simulink model "NULMPC_RAS"  (R2024a)
settings: Solver=FixedStepAuto  StartTime=0.0  StopTime=10  FixedStep=Ts  RelTol=1e-3
values from neighbouring files (symbols this model uses):
  alpha_o = 1/(ms) + 1/(mu)    [nulmpc.m]
  bs = 7.5    [initparams.m]
  bus = 5    [initparams.m]
  delta_Fc_max = 1000*Ts    (= 10)    [initparams.m]
  delta_Fc_min = -1000*Ts    (= -10)    [initparams.m]
  E = 1    [nmpc.m]    (also in nulmpc.m = 5)
  Fc_max = 15    [initparams.m]
  Fc_min = -15    [initparams.m]
  Hc = 1    [initparams.m]
  ks = 900    [initparams.m]
  kus = kt    (= 2500)    [initparams.m]
  ms = 2.45    [initparams.m]
  mus = mu    (= 1)    [initparams.m]
  n_max = 0.05    [initparams.m]
  n_min = -0.05    [initparams.m]
  Q_n = 10000    [nmpc.m]    (also in nulmpc.m = 1000)
  Q_ndot = 100    [nmpc.m]    (also in nulmpc.m = 5)
  R = 10    [nmpc.m]    (also in nulmpc.m)
  Ts = 0.01    [initparams.m]
  z1_dot_init = 0    [initparams.m]
  z1_init = 0.005    [initparams.m]
  z2_dot_init = 0    [initparams.m]
  z2_init = 0    [initparams.m]
libraries: simulink x1, mpclib x1
settings Model: Creator=aidan  LastModifiedBy=aidan
settings DebuggingCC: UnderSpecifiedDimensionMsg=warning
settings HardwareCC: ProdHWDeviceType=AMD->x86-64 (Windows64)

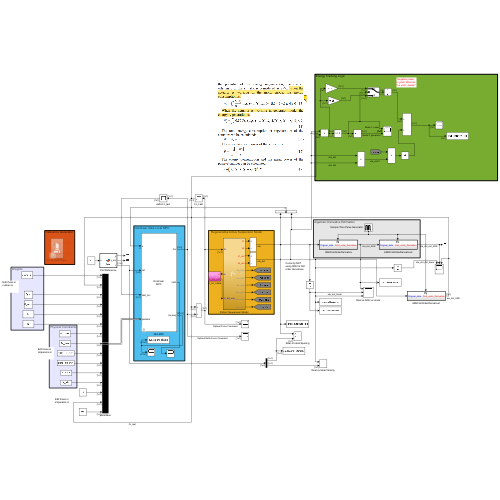
[thumbnail: Simulink's stored preview of the top-level diagram]
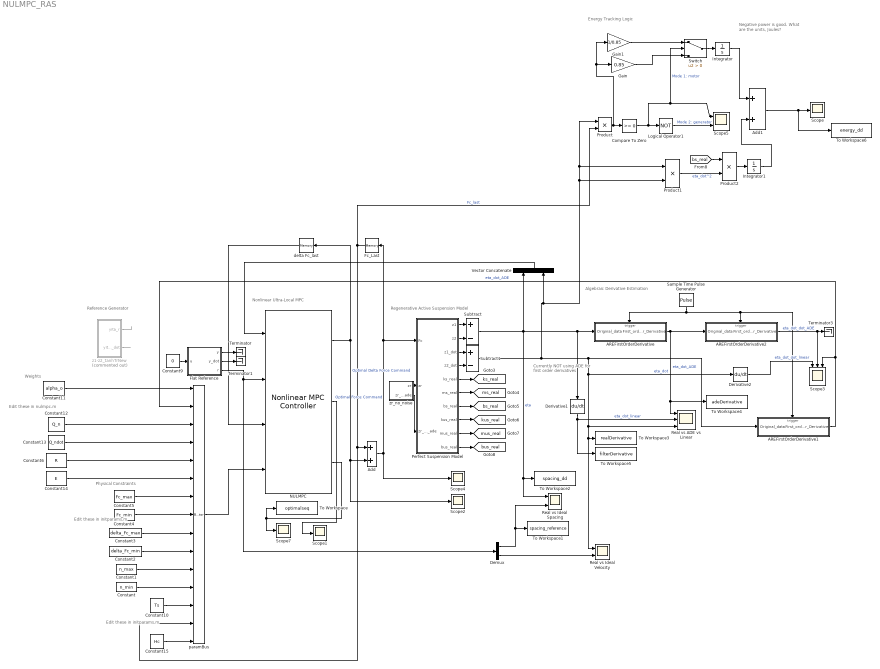
== system NULMPC_RAS ==
  note: Edit these in nulmpc.m
  note: Currently NOT using ADE for first order derivatives
  note: Nonlinear Ultra-Local MPC
  note: Energy Tracking Logic
  note: Regenerative Active Suspension Model
  note: Reference Generator
  note: Algebraic Derivative Estimation
  note: Weights
  note: Physical Constraints
  note: Negative power is good. What are the units, Joules?
  note: Edit these in initparams.m
  note: Edit these in initparams.m
  AREFirstOrderDerivative : Subsystem  TreatAsAtomicUnit=on
  AREFirstOrderDerivative1 : Subsystem  TreatAsAtomicUnit=on
  AREFirstOrderDerivative2 : Subsystem  TreatAsAtomicUnit=on
  Add : Sum
  Add1 : Sum
  Compare To Zero : simulink/Logic and Bit Operations/Compare To Zero  relop=>=  OutDataTypeStr=boolean
  Constant : Constant  Value=n_min
  Constant1 : Constant  Value=n_max
  Constant10 : Constant  Value=Ts
  Constant11 : Constant  Value=alpha_o
  Constant12 : Constant  Value=Q_n
  Constant13 : Constant  Value=Q_ndot
  Constant14 : Constant  Value=E
  Constant15 : Constant  Value=Hc
  Constant2 : Constant  Value=delta_Fc_min
  Constant3 : Constant  Value=delta_Fc_max
  Constant4 : Constant  Value=Fc_min
  Constant5 : Constant  Value=Fc_max
  Constant6 : Constant  Value=R
  Constant9 : Constant  Value=0
  Demux : Demux  Outputs=2
  Derivative1 : Derivative
  Derivative2 : Derivative
  Fc_Last : Memory  InheritSampleTime=on
  Flat Reference : MATLAB Function  TreatAsAtomicUnit=on
  Gain : Gain  Gain=0.85
  Gain1 : Gain  Gain=1/0.85
  Integrator : Integrator
  Integrator1 : Integrator
  Logical Operator1 : Logic  Operator=NOT  AllPortsSameDT=off  OutDataTypeStr=boolean
  NULMPC : mpclib/Nonlinear MPC Controller  nlmpcobj=nulmpcobj  UseObjectTs=on  UseMEX=off  md_enabled=off  mvtarget_enabled=off  param_enabled=on  cost_enabled=on  mvseq_enabled=on  stateseq_enabled=off  ovseq_enabled=off  slack_enabled=off  status_enabled=off  ov_min=off  ov_max=off  mv_min=off  mv_max=off  mvrate_min=off  mvrate_max=off  state_min=off  state_max=off  ov_weight=off  mv_weight=off  mvrate_weight=off  ecr_weight=off  nlp_initialize=off
  Perfect Suspension Model : Subsystem
  Product : Product
  Product1 : Product
  Product2 : Product
  Real vs ADE vs Linear : Scope  NumInputPorts=3
  Real vs Ideal Spacing : Scope  NumInputPorts=2
  Real vs Ideal Velocity : Scope  NumInputPorts=2
  Sample Time Pulse Generator : DiscretePulseGenerator  PulseType=Time based  Period=Ts*2  PulseWidth=50
  Scope{,1..2,4,7} (5 alike) : Scope
  Scope3 : Scope  NumInputPorts=3
  Scope5 : Scope  NumInputPorts=2
  Subtract : Sum  Inputs=+-
  Subtract1 : Sum  Inputs=+-
  Switch : Switch  Criteria=u2 > Threshold  SaturateOnIntegerOverflow=off  InputSameDT=off
  Terminator : Terminator
  Terminator1 : Terminator
  Terminator3 : Terminator
  To Workspace : ToWorkspace  VariableName=optimalseq  SaveFormat=Timeseries  SampleTime=-1
  To Workspace1 : ToWorkspace  VariableName=spacing_reference  SaveFormat=Timeseries  SampleTime=-1
  To Workspace2 : ToWorkspace  VariableName=spacing_dd  SaveFormat=Timeseries  SampleTime=-1
  To Workspace3 : ToWorkspace  VariableName=realDerivative  SaveFormat=Timeseries  SampleTime=-1
  To Workspace4 : ToWorkspace  VariableName=adeDerivative  SaveFormat=Timeseries  SampleTime=-1
  To Workspace5 : ToWorkspace  VariableName=filterDerivative  SaveFormat=Timeseries  SampleTime=-1
  To Workspace6 : ToWorkspace  VariableName=energy_dd  SaveFormat=Timeseries  SampleTime=-1
  Vector Concatenate : Concatenate
  delta Fc_last : Memory  InheritSampleTime=on
  paramBus : BusCreator  Inputs=15  OutDataTypeStr=Bus: paramBus  NonVirtualBus=on
      settings: InheritFromInputs=off
  "z1-z2_tanhTrNew " : Subsystem  Commented=on
  zr_no_noise : Subsystem
  tag scope: bs_real=global, bus_real=global, ks_real=global, kus_real=global, ms_real=global, mus_real=global
  wires:
  Constant5/1 -> paramBus/7
  Constant4/1 -> paramBus/8
  Constant3/1 -> paramBus/9
  Constant2/1 -> paramBus/10
  Constant1/1 -> paramBus/11
  Constant/1 -> paramBus/12
  Constant6/1 -> paramBus/5
  NULMPC/1 -> delta Fc_last/1, Scope2/1, Add/2  "Optimal Delta Force Command"
  Perfect Suspension Model/5(ks_real) -> [ks_real]
  Perfect Suspension Model/6(ms_real) -> [ms_real]
  Perfect Suspension Model/7(bs_real) -> [bs_real]
  Perfect Suspension Model/8(kus_real) -> [kus_real]
  Perfect Suspension Model/9(mus_real) -> [mus_real]
  Perfect Suspension Model/10(bus_real) -> [bus_real]
  Perfect Suspension Model/3(z1_dot) -> Subtract1/1
  Perfect Suspension Model/4(z2_dot) -> Subtract1/2
  Perfect Suspension Model/2(z2) -> Subtract/2
  Perfect Suspension Model/1(z1) -> Subtract/1
  Sample Time Pulse Generator/1 -> AREFirstOrderDerivative1/Trigger, AREFirstOrderDerivative2/Trigger, AREFirstOrderDerivative/Trigger
  Fc_Last/1 -> paramBus/14, Add/1, Product/2  "Fc_last"
  AREFirstOrderDerivative/1(First_order_Derivative) -> AREFirstOrderDerivative2/1(Original_data), To Workspace4/1, Real vs ADE vs Linear/1  "eta_dot_ADE"
  AREFirstOrderDerivative2/1(First_order_Derivative) -> Scope3/2, Terminator3/1  "eta_dot_dot_ADE"
  Vector Concatenate/1 -> NULMPC/1
  Constant13/1 -> paramBus/4
  Constant12/1 -> paramBus/3
  Add/1 -> Scope4/1, Perfect Suspension Model/1(Fc), Fc_Last/1  "Optimal Force Command"
  Derivative1/1 -> To Workspace5/1, Real vs ADE vs Linear/2  "eta_dot_linear"
  Derivative2/1 -> Scope3/1  "eta_dot_dot_linear"
  Subtract/1 -> Real vs Ideal Spacing/1, To Workspace2/1, Vector Concatenate/1, AREFirstOrderDerivative/1(Original_data), Derivative1/1  "eta"
  zr_no_noise/1(zr) -> Perfect Suspension Model/2(zr)
  Constant9/1 -> Flat Reference/1(u)
  "z1-z2_tanhTrNew "/2(yitar_dot) -> ?
  "z1-z2_tanhTrNew "/1(yita_r) -> ?
  Flat Reference/2(y_dot) -> Terminator1/1
  Flat Reference/1(y) -> Terminator/1
  paramBus/1 -> NULMPC/4
  Constant11/1 -> paramBus/1
  Constant14/1 -> paramBus/6
  delta Fc_last/1 -> NULMPC/3
  Constant10/1 -> paramBus/13
  Flat Reference/3(r) -> Demux/1, NULMPC/2
  Constant15/1 -> paramBus/15
  Demux/1 -> Real vs Ideal Spacing/2, To Workspace1/1
  Demux/2 -> Real vs Ideal Velocity/2
  Logical Operator1/1 -> Scope5/2  "Mode 2: generator"
  Compare To Zero/1 -> Switch/2, Scope5/1, Logical Operator1/1  "Mode 1: motor"
  NULMPC/2 -> Scope1/1
  NULMPC/3 -> Scope7/1, To Workspace/1
  Product/1 -> Gain/1, Gain1/1, Compare To Zero/1
  Switch/1 -> Integrator/1
  Gain/1 -> Switch/3
  Gain1/1 -> Switch/1
  AREFirstOrderDerivative1/1(First_order_Derivative) -> paramBus/2, Scope3/3  "eta_dot_ADE"
  zr_no_noise/2(zr_dot_ade) -> Perfect Suspension Model/3(zr_dot_ade)
  Subtract1/1 -> Vector Concatenate/2, Product/1, Product1/1, Product1/2, AREFirstOrderDerivative1/1(Original_data), Real vs Ideal Velocity/1, To Workspace3/1, Real vs ADE vs Linear/3, Derivative2/1  "eta_dot"
  Integrator1/1 -> Add1/2
  Product2/1 -> Integrator1/1
  Product1/1 -> Product2/2  "eta_dot^2"
  [bs_real] -> Product2/1
  Integrator/1 -> Add1/1
  Add1/1 -> Scope/1, To Workspace6/1

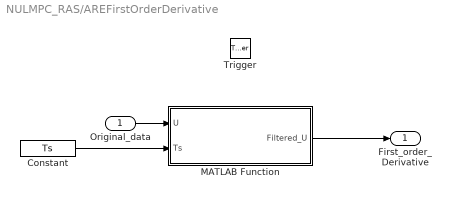
== system NULMPC_RAS/AREFirstOrderDerivative ==
  Original_data : Inport
  Trigger : TriggerPort  TriggerType=either  VariantControl=Variant  ZeroCross=off  PortDimensions=1
  Constant : Constant  Value=Ts
  MATLAB Function : MATLAB Function  TreatAsAtomicUnit=on
  First_order_Derivative : Outport  VectorParamsAs1DForOutWhenUnconnected=off
  wires:
  Constant/1 -> MATLAB Function/2(Ts)
  MATLAB Function/1(Filtered_U) -> First_order_Derivative/1
  Original_data/1 -> MATLAB Function/1(U)

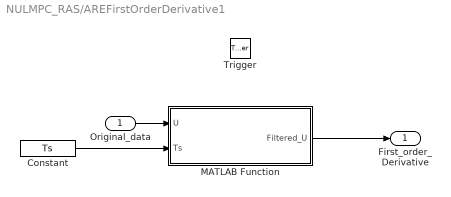
== system NULMPC_RAS/AREFirstOrderDerivative1 ==
  Original_data : Inport
  Trigger : TriggerPort  TriggerType=either  VariantControl=Variant  ZeroCross=off  PortDimensions=1
  Constant : Constant  Value=Ts
  MATLAB Function : MATLAB Function  TreatAsAtomicUnit=on
  First_order_Derivative : Outport  VectorParamsAs1DForOutWhenUnconnected=off
  wires:
  Constant/1 -> MATLAB Function/2(Ts)
  MATLAB Function/1(Filtered_U) -> First_order_Derivative/1
  Original_data/1 -> MATLAB Function/1(U)

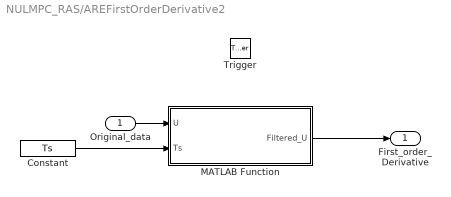
== system NULMPC_RAS/AREFirstOrderDerivative2 ==
  Original_data : Inport
  Trigger : TriggerPort  TriggerType=either  VariantControl=Variant  ZeroCross=off  PortDimensions=1
  Constant : Constant  Value=Ts
  MATLAB Function : MATLAB Function  TreatAsAtomicUnit=on
  First_order_Derivative : Outport  VectorParamsAs1DForOutWhenUnconnected=off
  wires:
  Constant/1 -> MATLAB Function/2(Ts)
  MATLAB Function/1(Filtered_U) -> First_order_Derivative/1
  Original_data/1 -> MATLAB Function/1(U)

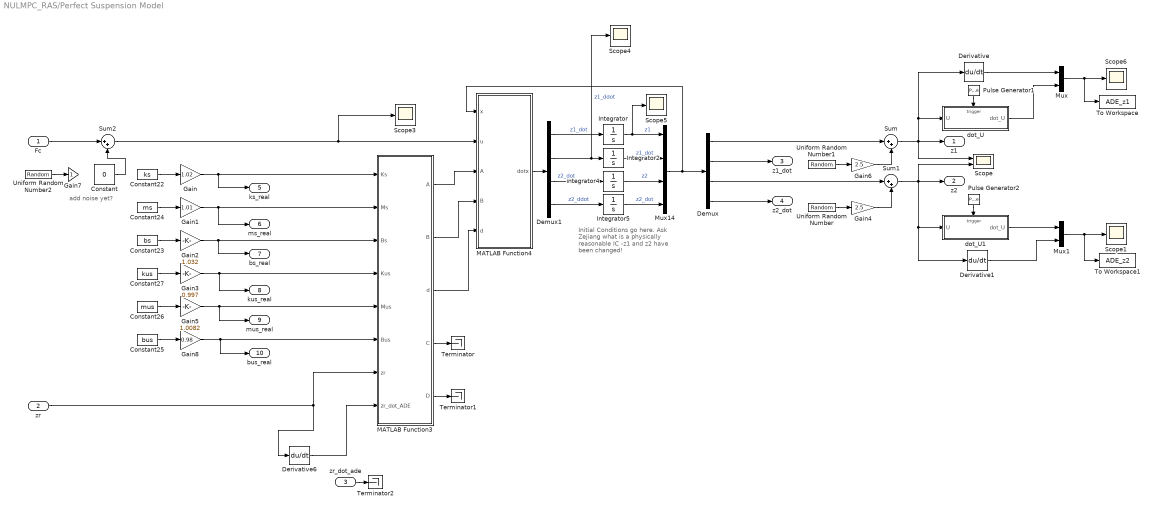
== system NULMPC_RAS/Perfect Suspension Model ==
  note: Initial Conditions go here. Ask Zejiang what is a physically reasonable IC
      |
      | -z1 and z2 have been changed!
  note: add noise yet?
  Fc : Inport
  zr : Inport  Port=2
  zr_dot_ade : Inport  Port=3
  Constant : Constant  Value=0
  Constant22 : Constant  Value=ks
  Constant23 : Constant  Value=bs
  Constant24 : Constant  Value=ms
  Constant25 : Constant  Value=bus
  Constant26 : Constant  Value=mus
  Constant27 : Constant  Value=kus
  Demux : Demux
  Demux1 : Demux
  Derivative : Derivative
  Derivative1 : Derivative
  Derivative6 : Derivative
  Gain : Gain  Gain=1.02
  Gain1 : Gain  Gain=1.01
  Gain2 : Gain  Gain=1.032
  Gain3 : Gain  Gain=0.997
  Gain4 : Gain  Gain=2.5
  Gain5 : Gain  Gain=1.0082
  Gain6 : Gain  Gain=2.5
  Gain7 : Gain
  Gain8 : Gain  Gain=0.98
  Integrator : Integrator  InitialCondition=z1_init
  Integrator2 : Integrator  InitialCondition=z1_dot_init
  Integrator4 : Integrator  InitialCondition=z2_init
  Integrator5 : Integrator  InitialCondition=z2_dot_init
  MATLAB Function3 : MATLAB Function  TreatAsAtomicUnit=on
  MATLAB Function4 : MATLAB Function  TreatAsAtomicUnit=on
  Mux : Mux  Inputs=2
  Mux1 : Mux  Inputs=2
  Mux14 : Mux
  Pulse Generator1 : DiscretePulseGenerator  PulseType=Time based  Period=Ts*2  PulseWidth=50
  Pulse Generator2 : DiscretePulseGenerator  PulseType=Time based  Period=Ts*2  PulseWidth=50
  Scope : Scope  NumInputPorts=2
  Scope{1,3..6} (5 alike) : Scope
  Sum : Sum  Inputs=|++
  Sum1 : Sum  Inputs=|++
  Sum2 : Sum  Inputs=|++
  Terminator : Terminator
  Terminator1 : Terminator
  Terminator2 : Terminator
  To Workspace : ToWorkspace  VariableName=ADE_z1  SampleTime=-1
  To Workspace1 : ToWorkspace  VariableName=ADE_z2  SampleTime=-1
  Uniform Random Number : UniformRandomNumber  Minimum=-1e-6  Maximum=1e-6  Seed=244334  SampleTime=Ts
  Uniform Random Number1 : UniformRandomNumber  Minimum=-1e-6  Maximum=1e-6  Seed=7  SampleTime=Ts
  Uniform Random Number2 : UniformRandomNumber  Minimum=-5e-3  Maximum=5e-3  Seed=89757  SampleTime=Ts
  dot_U : Subsystem  TreatAsAtomicUnit=on
  dot_U1 : Subsystem  TreatAsAtomicUnit=on
  z1 : Outport
  z2 : Outport  Port=2
  z1_dot : Outport  Port=3
  z2_dot : Outport  Port=4
  ks_real : Outport  Port=5
  ms_real : Outport  Port=6
  bs_real : Outport  Port=7
  kus_real : Outport  Port=8
  mus_real : Outport  Port=9
  bus_real : Outport  Port=10
  wires:
  Constant23/1 -> Gain2/1
  MATLAB Function3/4(C) -> Terminator/1
  Demux1/1 -> Integrator/1  "z1_dot"
  zr/1 -> MATLAB Function3/7(zr), Derivative6/1
  Integrator5/1 -> Mux14/4  "z2_dot"
  Demux1/2 -> Scope4/1, Integrator2/1  "z1_ddot"
  Gain2/1 -> bs_real/1, MATLAB Function3/3(Bs)
  Constant27/1 -> Gain3/1
  Gain3/1 -> kus_real/1, MATLAB Function3/4(Kus)
  Constant24/1 -> Gain1/1
  Constant25/1 -> Gain8/1
  Demux1/4 -> Integrator5/1  "z2_ddot"
  MATLAB Function4/1(dotx) -> Demux1/1
  Integrator4/1 -> Mux14/3  "z2"
  Integrator/1 -> Scope5/1, Mux14/1  "z1"
  Constant26/1 -> Gain5/1
  Gain8/1 -> bus_real/1, MATLAB Function3/6(Bus)
  MATLAB Function3/2(B) -> MATLAB Function4/4(B)
  Constant22/1 -> Gain/1
  Demux1/3 -> Integrator4/1  "z2_dot"
  Gain5/1 -> mus_real/1, MATLAB Function3/5(Mus)
  MATLAB Function3/5(D) -> Terminator1/1
  Integrator2/1 -> Mux14/2  "z1_dot"
  Gain1/1 -> ms_real/1, MATLAB Function3/2(Ms)
  Gain/1 -> ks_real/1, MATLAB Function3/1(Ks)
  MATLAB Function3/1(A) -> MATLAB Function4/3(A)
  Mux14/1 -> Demux/1, MATLAB Function4/1(x)
  MATLAB Function3/3(d) -> MATLAB Function4/5(d)
  Demux/2 -> z1_dot/1
  Demux/4 -> z2_dot/1
  Gain4/1 -> Sum1/2
  Uniform Random Number/1 -> Gain4/1
  Sum/1 -> Scope/1, Derivative/1, dot_U/1(U), z1/1
  Demux/1 -> Sum/1
  Demux/3 -> Sum1/1
  Uniform Random Number1/1 -> Gain6/1
  Gain6/1 -> Sum/2
  dot_U/1(dot_U) -> Mux/2
  Pulse Generator1/1 -> dot_U/Trigger
  Derivative/1 -> Mux/1
  Pulse Generator2/1 -> dot_U1/Trigger
  Sum1/1 -> Scope/2, Derivative1/1, dot_U1/1(U), z2/1
  dot_U1/1(dot_U) -> Mux1/1
  Derivative1/1 -> Mux1/2
  Sum2/1 -> Scope3/1, MATLAB Function4/2(u)
  Fc/1 -> Sum2/1
  Uniform Random Number2/1 -> Gain7/1
  Mux/1 -> To Workspace/1, Scope6/1
  Mux1/1 -> Scope1/1, To Workspace1/1
  Constant/1 -> Sum2/2
  zr_dot_ade/1 -> Terminator2/1
  Derivative6/1 -> MATLAB Function3/8(zr_dot_ADE)

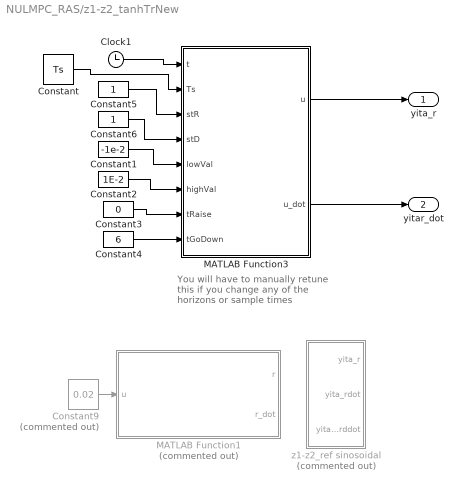
== system NULMPC_RAS/z1-z2_tanhTrNew  ==
  note: You will have to manually retune this if you change any of the horizons or sample times
  Clock1 : Clock
  Constant : Constant  Value=Ts
  Constant1 : Constant  Value=-1e-2
  Constant2 : Constant  Value=1E-2
  Constant3 : Constant  Value=0
  Constant4 : Constant  Value=6
  Constant5 : Constant
  Constant6 : Constant
  Constant9 : Constant  Commented=on  Value=0.02
  MATLAB Function1 : MATLAB Function  Commented=on  TreatAsAtomicUnit=on
  MATLAB Function3 : MATLAB Function  TreatAsAtomicUnit=on
  z1-z2_ref sinosoidal : Subsystem  Commented=on
  yita_r : Outport
  yitar_dot : Outport  Port=2
  wires:
  Constant5/1 -> MATLAB Function3/3(stR)
  Constant4/1 -> MATLAB Function3/8(tGoDown)
  Constant3/1 -> MATLAB Function3/7(tRaise)
  Clock1/1 -> MATLAB Function3/1(t)
  Constant6/1 -> MATLAB Function3/4(stD)
  MATLAB Function3/1(u) -> yita_r/1
  Constant1/1 -> MATLAB Function3/5(lowVal)
  Constant2/1 -> MATLAB Function3/6(highVal)
  MATLAB Function3/2(u_dot) -> yitar_dot/1
  Constant/1 -> MATLAB Function3/2(Ts)
  Constant9/1 -> MATLAB Function1/1(u)

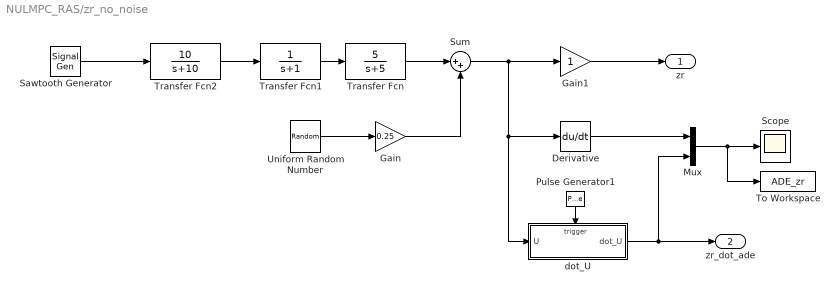
== system NULMPC_RAS/zr_no_noise ==
  Derivative : Derivative
  Gain : Gain  Gain=0.25
  Gain1 : Gain
  Mux : Mux  Inputs=2
  Pulse Generator1 : DiscretePulseGenerator  PulseType=Time based  Period=Ts*2  PulseWidth=50
  Sawtooth Generator : SignalGenerator  WaveForm=sawtooth  Amplitude=3.5e-2
  Scope : Scope
  Sum : Sum  Inputs=|++
  To Workspace : ToWorkspace  VariableName=ADE_zr  SampleTime=-1
  Transfer Fcn : TransferFcn  Numerator=[5]  Denominator=[1 5]
  Transfer Fcn1 : TransferFcn  Denominator=[1 1]
  Transfer Fcn2 : TransferFcn  Numerator=[10]  Denominator=[1 10]
  Uniform Random Number : UniformRandomNumber  Minimum=-1e-6  Maximum=1e-6  Seed=122334  SampleTime=Ts
  dot_U : Subsystem  TreatAsAtomicUnit=on
  zr : Outport
  zr_dot_ade : Outport  Port=2
  wires:
  Transfer Fcn2/1 -> Transfer Fcn1/1
  Transfer Fcn/1 -> Sum/1
  Sawtooth Generator/1 -> Transfer Fcn2/1
  Transfer Fcn1/1 -> Transfer Fcn/1
  Uniform Random Number/1 -> Gain/1
  Gain/1 -> Sum/2
  Pulse Generator1/1 -> dot_U/Trigger
  Derivative/1 -> Mux/1
  dot_U/1(dot_U) -> zr_dot_ade/1, Mux/2
  Mux/1 -> To Workspace/1, Scope/1
  Sum/1 -> dot_U/1(U), Derivative/1, Gain1/1
  Gain1/1 -> zr/1

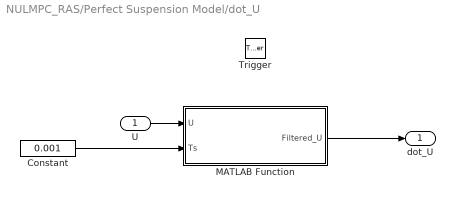
== system NULMPC_RAS/Perfect Suspension Model/dot_U ==
  U : Inport
  Trigger : TriggerPort  TriggerType=either  VariantControl=Variant  ZeroCross=off  PortDimensions=1
  Constant : Constant  Value=0.001
  MATLAB Function : MATLAB Function  TreatAsAtomicUnit=on
  dot_U : Outport  VectorParamsAs1DForOutWhenUnconnected=off
  wires:
  Constant/1 -> MATLAB Function/2(Ts)
  MATLAB Function/1(Filtered_U) -> dot_U/1
  U/1 -> MATLAB Function/1(U)

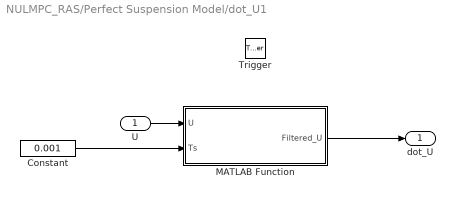
== system NULMPC_RAS/Perfect Suspension Model/dot_U1 ==
  U : Inport
  Trigger : TriggerPort  TriggerType=either  VariantControl=Variant  ZeroCross=off  PortDimensions=1
  Constant : Constant  Value=0.001
  MATLAB Function : MATLAB Function  TreatAsAtomicUnit=on
  dot_U : Outport  VectorParamsAs1DForOutWhenUnconnected=off
  wires:
  U/1 -> MATLAB Function/1(U)
  MATLAB Function/1(Filtered_U) -> dot_U/1
  Constant/1 -> MATLAB Function/2(Ts)

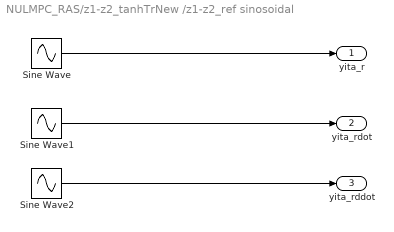
== system NULMPC_RAS/z1-z2_tanhTrNew /z1-z2_ref sinosoidal ==
  Sine Wave : Sin  Amplitude=1e-2  Frequency=2*pi/5  SampleTime=0
  Sine Wave1 : Sin  Amplitude=1e-2*2*pi/5  Frequency=2*pi/5  Phase=pi/2  SampleTime=0
  Sine Wave2 : Sin  Amplitude=-1e-2*(2*pi/5)^2  Frequency=2*pi/5  SampleTime=0
  yita_r : Outport
  yita_rdot : Outport  Port=2
  yita_rddot : Outport  Port=3
  wires:
  Sine Wave/1 -> yita_r/1
  Sine Wave1/1 -> yita_rdot/1
  Sine Wave2/1 -> yita_rddot/1

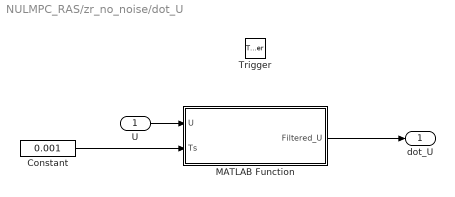
== system NULMPC_RAS/zr_no_noise/dot_U ==
  U : Inport
  Trigger : TriggerPort  TriggerType=either  VariantControl=Variant  ZeroCross=off  PortDimensions=1
  Constant : Constant  Value=0.001
  MATLAB Function : MATLAB Function  TreatAsAtomicUnit=on
  dot_U : Outport  VectorParamsAs1DForOutWhenUnconnected=off
  wires:
  Constant/1 -> MATLAB Function/2(Ts)
  MATLAB Function/1(Filtered_U) -> dot_U/1
  U/1 -> MATLAB Function/1(U)

== matlab function NULMPC_RAS/AREFirstOrderDerivative2/MATLAB Function ==
  data: U input; Filtered_U output; Ts input
function Filtered_U = buffer(U,Ts)
    N = 8; %6
    %Ts = 0.01;
    persistent y;
    if isempty(y)
        y=zeros(N+1,1);
    end

    y = [U;y(1:end-1)];
    T = Ts*N;
    P = zeros(1,N+1);
    P_alpha = P;
    for k = 1:N+1
        tao_k = (k-1)*Ts;
        P(k) = T-2*tao_k;
        if((k==1)||(k==N+1))
            P_alpha(k) = P(k)*Ts/2;
        else
            P_alpha(k) = P(k)*Ts;
        end
    end
    
    Filtered_U = P_alpha*y*6/(T^3);

end

== matlab function NULMPC_RAS/Perfect Suspension Model/MATLAB Function4 ==
  data: x input; dotx output; u input; A input; B input; d input
function dotx  = Susp_System(x, u, A, B, d)
    
    dotx = A*x + B*u + d;
    %y = C*x + D*u;
end

== matlab function NULMPC_RAS/AREFirstOrderDerivative/MATLAB Function ==
  data: U input; Filtered_U output; Ts input
function Filtered_U = buffer(U,Ts)
    % was 12
    N = 8;
    persistent y;
    if isempty(y)
        y=zeros(N+1,1);
    end

    y = [U;y(1:end-1)];
    T = Ts*N;
    P = zeros(1,N+1);
    P_alpha = P;
    for k = 1:N+1
        tao_k = (k-1)*Ts;
        P(k) = T-2*tao_k;
        if((k==1)||(k==N+1))
            P_alpha(k) = P(k)*Ts/2;
        else
            P_alpha(k) = P(k)*Ts;
        end
    end
    
    Filtered_U = P_alpha*y*6/(T^3);

end

== matlab function NULMPC_RAS/Perfect Suspension Model/MATLAB Function3 ==
  data: Ks input; A output; Ms input; Bs input; Kus input; Mus input; Bus input; zr input; zr_dot_ADE input; B output; d output; C output; D output
function [A, B, d, C, D] = Syst(Ks, Ms, Bs, Kus, Mus, Bus, zr, zr_dot_ADE)
    A = [    0,      1,             0,              0; 
        -Ks/Ms, -Bs/Ms,         Ks/Ms,          Bs/Ms; 
             0,      0,             0,              1; 
        Ks/Mus, Bs/Mus, -(Kus+Ks)/Mus, -(Bus+Bs)/Mus];
 
    
    B = [0; 1/Ms; 0; -1/Mus];
    
    
    d = [0;    0; 0;  Kus/Mus*zr + Bus/Mus*zr_dot_ADE];
   
    
    C = [    1,      0,    -1,     0;
        -Ks/Ms, -Bs/Ms, Ks/Ms, Bs/Ms];
    
    D = [0; 1/Ms];
    
    
end

== matlab function NULMPC_RAS/zr_no_noise/dot_U/MATLAB Function ==
  data: U input; Filtered_U output; Ts input
function Filtered_U = buffer(U,Ts)
    N = 10;
    %Ts = 0.001;
    persistent y;
    if isempty(y)
        y=zeros(N+1,1);
    end

    y = [U;y(1:end-1)];
    T = Ts*N;
    P = zeros(1,N+1);
    P_alpha = P;
    for k = 1:N+1
        tao_k = (k-1)*Ts;
        P(k) = T-2*tao_k;
        if((k==1)||(k==N+1))
            P_alpha(k) = P(k)*Ts/2;
        else
            P_alpha(k) = P(k)*Ts;
        end
    end
    
    Filtered_U = P_alpha*y*6/(T^3);

end

== matlab function NULMPC_RAS/AREFirstOrderDerivative1/MATLAB Function ==
  data: U input; Filtered_U output; Ts input
function Filtered_U = buffer(U,Ts)
    % was 12
    N = 4;
    persistent y;
    if isempty(y)
        y=zeros(N+1,1);
    end

    y = [U;y(1:end-1)];
    T = Ts*N;
    P = zeros(1,N+1);
    P_alpha = P;
    for k = 1:N+1
        tao_k = (k-1)*Ts;
        P(k) = T-2*tao_k;
        if((k==1)||(k==N+1))
            P_alpha(k) = P(k)*Ts/2;
        else
            P_alpha(k) = P(k)*Ts;
        end
    end
    
    Filtered_U = P_alpha*y*6/(T^3);

end

== matlab function NULMPC_RAS/Perfect Suspension Model/dot_U/MATLAB Function ==
  data: U input; Filtered_U output; Ts input
function Filtered_U = buffer(U,Ts)
    N = 10;
    %Ts = 0.001;
    persistent y;
    if isempty(y)
        y=zeros(N+1,1);
    end

    y = [U;y(1:end-1)];
    T = Ts*N;
    P = zeros(1,N+1);
    P_alpha = P;
    for k = 1:N+1
        tao_k = (k-1)*Ts;
        P(k) = T-2*tao_k;
        if((k==1)||(k==N+1))
            P_alpha(k) = P(k)*Ts/2;
        else
            P_alpha(k) = P(k)*Ts;
        end
    end
    
    Filtered_U = P_alpha*y*6/(T^3);

end

== matlab function NULMPC_RAS/Perfect Suspension Model/dot_U1/MATLAB Function ==
  data: U input; Filtered_U output; Ts input
function Filtered_U = buffer(U,Ts)
    N = 10;
    %Ts = 0.001;
    persistent y;
    if isempty(y)
        y=zeros(N+1,1);
    end

    y = [U;y(1:end-1)];
    T = Ts*N;
    P = zeros(1,N+1);
    P_alpha = P;
    for k = 1:N+1
        tao_k = (k-1)*Ts;
        P(k) = T-2*tao_k;
        if((k==1)||(k==N+1))
            P_alpha(k) = P(k)*Ts/2;
        else
            P_alpha(k) = P(k)*Ts;
        end
    end
    
    Filtered_U = P_alpha*y*6/(T^3);

end

== matlab function NULMPC_RAS/z1-z2_tanhTrNew /MATLAB Function1 ==
  data: u input; r output; r_dot output
function [r, r_dot]= constantReference(u)

r = u + zeros(20,1);
r_dot = zeros(20,1);

end

== matlab function NULMPC_RAS/Flat Reference ==
  data: u input; y output; y_dot output; r output
function [y, y_dot, r]= fcn(u)

y = u;
y_dot = 0;
% r = [y;y_dot];
r = [y,y_dot];

== matlab function NULMPC_RAS/z1-z2_tanhTrNew /MATLAB Function3 ==
  data: t input; Ts input; u output; stR input; stD input; lowVal input; highVal input; tRaise input; tGoDown input; u_dot output
function [u, u_dot] = tanhHatTr(t, Ts, stR, stD, lowVal, highVal,tRaise, tGoDown)
    % 20 is number of samples (equal to prediction horizon), 0.001 is equal
    % to Ts
    time_vec = t:Ts:t+30*Ts;
    u = zeros(30,1);
    u_dot =zeros(30,1);
    a = 0.5*(highVal-lowVal);

    for i=1:30
        phi = tanh(stR*((time_vec(i))-tRaise));
        psi = tanh(-stD*((time_vec(i))-tGoDown));

        u(i,1) = a .* (phi + psi) + lowVal;
        u_dot(i,1) = a .* (stR.*(1-phi.^2) - stD.*(1-psi.^2)); 
        %u_ddot = -2*a .* (stR.^2.*phi.*(1-phi.^2) + stD.^2.*psi.*(1-psi.^2))
    end

end
